simulink model "circuitTestSimulink_MDKTemplate_3DElectrical"  (R2024a)
settings: Solver=VariableStepAuto  StartTime=0.0  StopTime=1100e-9  FixedStep=1e-12  MaxStep=1e-10  RelTol=1e-2
undefined symbols (not defined in the file or in its folder): FMIKit
libraries: fl_lib x16, nesl_utility x10, ee_lib x4
settings Model: Creator=ezzbj2  LastModifiedBy=ezzbj2
settings SolverCC: ShapePreserveControl=EnableAll  ZeroCrossAlgorithm=Adaptive
settings RTWCC: GPUComputeCapability=3.5

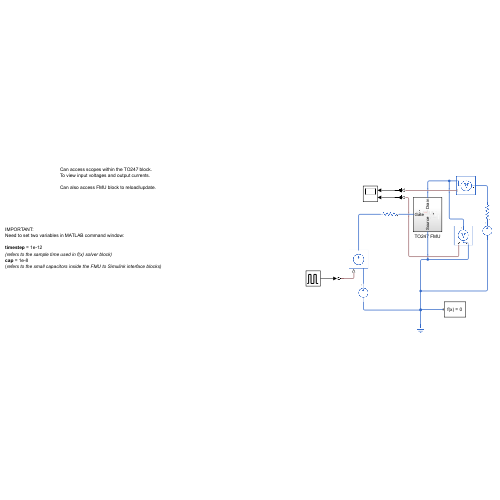
[thumbnail: Simulink's stored preview of the top-level diagram]
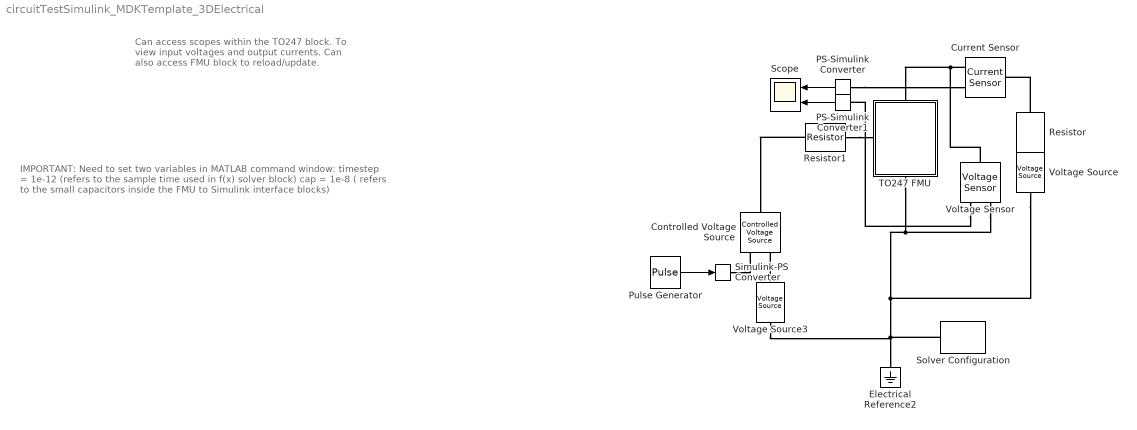
== system circuitTestSimulink_MDKTemplate_3DElectrical ==
  note: Can access scopes within the TO247 block.
      | To view input voltages and output currents.
      |
      | Can also access FMU block to reload/update.
  note: IMPORTANT:
      | Need to set two variables in MATLAB command window:
      |
      | timestep = 1e-12
      | (refers to the sample time used in f(x) solver block)
      | cap = 1e-8
      | ( refers to the small capacitors inside the FMU to Simulink interface blocks)
  Controlled Voltage Source : fl_lib/Electrical/Electrical Sources/Controlled Voltage Source
  Current Sensor : fl_lib/Electrical/Electrical Sensors/Current Sensor
  Electrical Reference2 : fl_lib/Electrical/Electrical Elements/Electrical Reference
  PS-Simulink Converter : nesl_utility/PS-Simulink Converter  PhysicalDomain=network_engine_domain  SubClassName=ps_output  LeftPortType=input  RightPortType=output  PseudoPeriodic=off  Frequencies=[]  VectorFormat=inherit  Unit=inherit  AffineConversion=off
  PS-Simulink Converter1 : nesl_utility/PS-Simulink Converter  PhysicalDomain=network_engine_domain  SubClassName=ps_output  LeftPortType=input  RightPortType=output  PseudoPeriodic=off  Frequencies=[]  VectorFormat=inherit  Unit=inherit  AffineConversion=off
  Pulse Generator : DiscretePulseGenerator  PulseType=Time based  Amplitude=15  Period=1000e-9  PulseWidth=50
  Resistor : ee_lib/Passive/Resistor  R=10 Ohm  enable_R_tol=ee.enum.toleranceApplication.none  R_tol=5  tol_distribution=ee.enum.toleranceDistribution.uniform  nSigma=4  enable_operating_limits=ee.enum.enable.no  operating_limit_action=ee.enum.passive.reportOpLim.warn  power_rating=1 W  max_working_voltage=100 V  enable_faults=ee.enum.enable.no  fault_action=simscape.enum.assert.action.none  R_faulted=inf Ohm  fault_trigger=ee.enum.faults.faultTrigger.temporal  t_fault=1 s  max_permissible_current=1 A  t_fail_on_current=1 s  noise_mode=ee.enum.sources.noise.Disabled  Tdevice=25 degC  sample_time=1e-3 s  repeatability=ee.enum.ic.repeatability.notRepeatable  user_seed=0  auto_seed=3499211588  faulted_specify=off  faulted_priority=None  faulted=0  power_derating_T1=70 degC  power_derating_T2=155 degC  operating_temperature_range_vec=[-50, 150] degC  alpha=3.93e-3 1/K  Tmeas=25 degC  thermal_mass=100 J/K  temperature_specify=off  temperature_priority=High  temperature=298.15 K  temperature_nominal_specify=off  temperature_nominal_value=1  temperature_nominal_unit=K
  Resistor1 : ee_lib/Passive/Resistor  R=2 Ohm  enable_R_tol=ee.enum.toleranceApplication.none  R_tol=5  tol_distribution=ee.enum.toleranceDistribution.uniform  nSigma=4  enable_operating_limits=ee.enum.enable.no  operating_limit_action=ee.enum.passive.reportOpLim.warn  power_rating=1 W  max_working_voltage=100 V  enable_faults=ee.enum.enable.no  fault_action=simscape.enum.assert.action.none  R_faulted=inf Ohm  fault_trigger=ee.enum.faults.faultTrigger.temporal  t_fault=1 s  max_permissible_current=1 A  t_fail_on_current=1 s  noise_mode=ee.enum.sources.noise.Disabled  Tdevice=25 degC  sample_time=1e-3 s  repeatability=ee.enum.ic.repeatability.notRepeatable  user_seed=0  auto_seed=3499211588  faulted_specify=off  faulted_priority=None  faulted=0  power_derating_T1=70 degC  power_derating_T2=155 degC  operating_temperature_range_vec=[-50, 150] degC  alpha=3.93e-3 1/K  Tmeas=25 degC  thermal_mass=100 J/K  temperature_specify=off  temperature_priority=High  temperature=298.15 K  temperature_nominal_specify=off  temperature_nominal_value=1  temperature_nominal_unit=K
  Scope : Scope  NumInputPorts=2
  Simulink-PS Converter : nesl_utility/Simulink-PS Converter  PhysicalDomain=network_engine_domain  SubClassName=ps_input  LeftPortType=input  RightPortType=output  PseudoPeriodic=off  Frequencies=[]  NoiseDistribution=none  NoiseParameters=[]  Unit=1  AffineConversion=off  FilteringAndDerivatives=provide  SimscapeFilterOrder=1  InputFilterTimeConstant=0.001  UdotUserProvided=0
  Solver Configuration : nesl_utility/Solver Configuration  PhysicalDomain=network_engine_domain  SubClassName=solver  LeftPortType=input  RightPortType=generic  Tones=[]  Harmonics=[]  SimulateNoise=off  Profile=off  UseLocalSampling=off  EnableSwitchedLinearOptims=on  FrequencyDomain=off  UseCCode=off  RelTol=0.001  AbsTol=0.001  MinStep=1e-09  ToWorkspace=off  RevertToSquareIcSolve=off  NumHomotopyIterations=100  PhasorMode=off  PhasorModeNumHarmonics=1  ConsistencySolver=NEWTON_XTOL_AFTER_FTOL  IndexReductionMethod=None  DoDC=on  ResidualTolerance=1e-09  ConsistencyTolSource=GLOBAL  ConsistencyAbsTol=0.001  ConsistencyRelTol=0.001  ConsistencyTolFactor=0.001  UseLocalSolver=off  LocalSolverChoice=NE_BACKWARD_EULER_ADVANCER  ResolveIndetEquations=on  FunctionEvalNumThread=1  LocalSolverSampleTime=timestep  DoFixedCost=off  MaxNonlinIter=30  MaxModeIter=2  ComputeImpulses=on  ImpulseIterations=2  LinearAlgebra=auto  LinearAlgebraNumThread=0  EquationFormulation=NE_TIME_EF  DelaysMemoryBudget=1024  AutomaticFiltering=off  FilteringTimeConstant=0.001  PartitionStorageMethod=EXHAUSTIVE  PartitionMemoryBudget=1024  PartitionMethod=ROBUST  MultibodyUseLocalSolver=off  MultibodyLocalSolverChoice=ODE1  MultibodyLocalSolverSampleTime=0.001
  TO247 FMU : Subsystem
      settings: PortSchema="{\"entries\":[{\"content\":{\"sides\":[{\"content\":{\"connectorIds\":[\"LConn1\"]},\"type\":\"ConnectorPlacement.EquallySpacedRectSide\",\"uuid\":\"1a7c621a-b2c4-44d6-8085-8acdfe65af3e\"},{\"content\":{\"side\":\"RIGHT\"},\"type\":\"ConnectorPlacement.EquallySpacedRectSide\",\"uuid\":\"009b5a79-97ab-42cc-83a0-e109b769c9f7\"},{\"content\":{\"connectorIds\":[\"LConn2\"],\"side\":\"TOP\"},\"type\":\"ConnectorPlacement.EquallySpacedRectSide\",\"uuid\":\"b2698f3e-d975-41db-922f-800e4c377170\"},{\"content\":{\"connectorIds\":[\"RConn1\"],\"side\":\"BOTTOM\"},\"type\":\"ConnectorPlacement.EquallySpacedRectSide\",\"uuid\":\"c87b7d4f-b69b-4cab-ae10-03d23c792008\"}]},\"type\":\"ConnectorPlacement.EquallySpacedConnector\",\"uuid\":\"776127ee-5564-4d8f-a192-88fd759918ca\"}],\"packageUris\":[\"http://schema.mathworks.com/mf0/Connector/R2020b\"],\"version\":\"1.0\"}"
  Voltage Sensor : fl_lib/Electrical/Electrical Sensors/Voltage Sensor
  Voltage Source : ee_lib/Sources/Voltage Source  dc_voltage=100 V  ac_voltage=0 V  ac_shift=0 rad  ac_frequency=60 Hz  noise_mode=ee.enum.sources.noise.Disabled  PSD=0 V^2/Hz  sample_time=1e-3 s  repeatability=ee.enum.sources.repeatability.NotRepeatable  user_seed=0  auto_seed=3890346746  i_specify=off  i_priority=None  i=0 A  i_nominal_specify=off  i_nominal_value=1  i_nominal_unit=A  v_specify=off  v_priority=None  v=0 V  v_nominal_specify=off  v_nominal_value=1  v_nominal_unit=V
  Voltage Source3 : ee_lib/Sources/Voltage Source  dc_voltage=0 V  ac_voltage=0 V  ac_shift=0 rad  ac_frequency=60 Hz  noise_mode=ee.enum.sources.noise.Disabled  PSD=0 V^2/Hz  sample_time=1e-3 s  repeatability=ee.enum.sources.repeatability.NotRepeatable  user_seed=0  auto_seed=3499211588  i_specify=off  i_priority=None  i=0 A  i_nominal_specify=off  i_nominal_value=1  i_nominal_unit=A  v_specify=off  v_priority=None  v=0 V  v_nominal_specify=off  v_nominal_value=1  v_nominal_unit=V
  wires:
  PS-Simulink Converter/1 -> Scope/1
  PS-Simulink Converter1/1 -> Scope/2
  Pulse Generator/1 -> Simulink-PS Converter/1
  connections:
  TO247 FMU/RConn1 -- Voltage Source/RConn1 -- Voltage Source3/RConn1 -- Electrical Reference2/LConn1 -- Solver Configuration/RConn1 -- Voltage Sensor/RConn2
  Current Sensor/RConn2 -- Voltage Sensor/LConn1 -- TO247 FMU/LConn2
  PS-Simulink Converter/LConn1 -- Current Sensor/RConn1
  Simulink-PS Converter/RConn1 -- Controlled Voltage Source/RConn1
  Voltage Source3/LConn1 -- Controlled Voltage Source/RConn2
  Voltage Sensor/RConn1 -- PS-Simulink Converter1/LConn1
  Resistor/RConn1 -- Voltage Source/LConn1
  Resistor/LConn1 -- Current Sensor/LConn1
  Resistor1/LConn1 -- TO247 FMU/LConn1
  Resistor1/RConn1 -- Controlled Voltage Source/LConn1

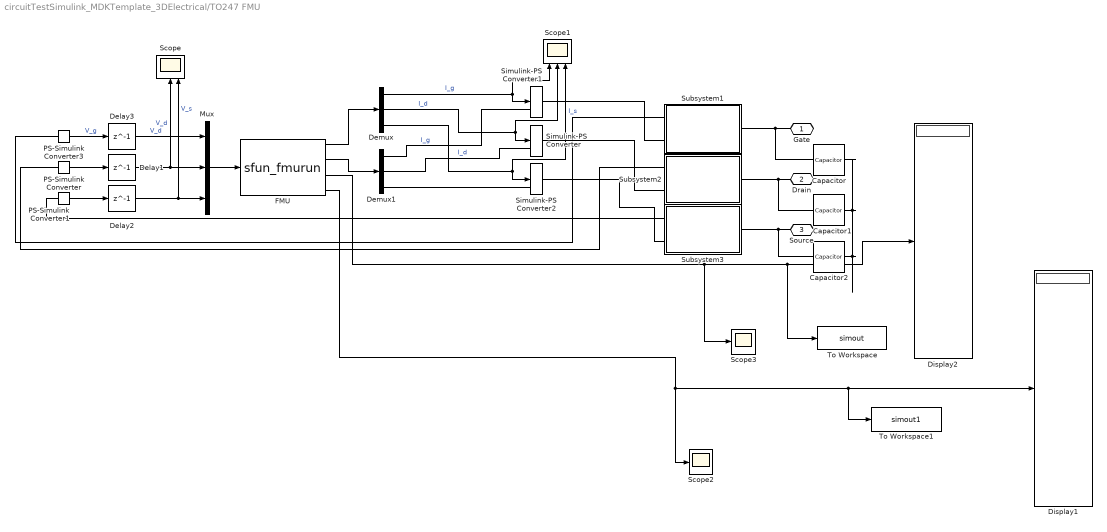
== system circuitTestSimulink_MDKTemplate_3DElectrical/TO247 FMU ==
  Capacitor : fl_lib/Electrical/Electrical Elements/Capacitor  c=1e-14 F  r=1e-6 Ohm  g=0 1/Ohm  i_specify=off  i_priority=None  i=0 A  i_nominal_specify=off  i_nominal_value=1  i_nominal_unit=A  v_specify=off  v_priority=None  v=0 V  v_nominal_specify=off  v_nominal_value=1  v_nominal_unit=V  vc_specify=off  vc_priority=High  vc=0 V  vc_nominal_specify=off  vc_nominal_value=1  vc_nominal_unit=V
  Capacitor1 : fl_lib/Electrical/Electrical Elements/Capacitor  c=1e-14 F  r=1e-6 Ohm  g=0 1/Ohm  i_specify=off  i_priority=None  i=0 A  i_nominal_specify=off  i_nominal_value=1  i_nominal_unit=A  v_specify=off  v_priority=None  v=0 V  v_nominal_specify=off  v_nominal_value=1  v_nominal_unit=V  vc_specify=off  vc_priority=High  vc=0 V  vc_nominal_specify=off  vc_nominal_value=1  vc_nominal_unit=V
  Capacitor2 : fl_lib/Electrical/Electrical Elements/Capacitor  c=1e-14 F  r=1e-6 Ohm  g=0 1/Ohm  i_specify=off  i_priority=None  i=0 A  i_nominal_specify=off  i_nominal_value=1  i_nominal_unit=A  v_specify=off  v_priority=None  v=0 V  v_nominal_specify=off  v_nominal_value=1  v_nominal_unit=V  vc_specify=off  vc_priority=High  vc=0 V  vc_nominal_specify=off  vc_nominal_value=1  vc_nominal_unit=V
  Delay1 : Delay  DelayLength=1
  Delay2 : Delay  DelayLength=1
  Delay3 : Delay  DelayLength=1
  Demux : Demux  Outputs=3
  Demux1 : Demux  Outputs=3
  Display1 : Display
  Display2 : Display
  FMU : S-Function  LoadFcn=FMIKit.setSFunctionParameters(gcb)  FunctionName=sfun_fmurun  Parameters=3.0 0 '{D773325B-AB94-4630-BF85-643EB24FCB80}' 'MDKCircuit_3DElectrical' FMIKit.getUnzipDirectory(gcb) 0 0 0 '' FMIKit.getSolverRelativeTolerance(bdroot(gcb)) -1 0 12 0 0 [3] [1.0] [2] [9] [3 3 16 12] [2 2 2 2] [10 24 13 11]  SFunctionDeploymentMode=off  EnableBusSupport=off
      settings: DeleteFcn=FMIKit.closeBlockDialog(gcbh)  ModelCloseFcn=FMIKit.closeBlockDialog(gcbh)  DestroyFcn=FMIKit.closeBlockDialog(gcbh)  OpenFcn=FMIKit.showBlockDialog(gcbh);  CloseFcn=FMIKit.closeBlockDialog(gcbh)  ParentCloseFcn=FMIKit.closeBlockDialog(gcbh)
      mask Help: eval('FMIKit.showBlockDialogHelp();')
      mask Display:
      | port_label('input', 1, 'u');
      | port_label('output', 1, 'y');
      | port_label('output', 2, 'dy');
      | port_label('output', 3, 'x_a');
      | port_label('output', 4, 'x_d');
  Mux : Mux  Inputs=3
  PS-Simulink Converter : nesl_utility/PS-Simulink Converter  PhysicalDomain=network_engine_domain  SubClassName=ps_output  LeftPortType=input  RightPortType=output  PseudoPeriodic=off  Frequencies=[]  VectorFormat=inherit  Unit=inherit  AffineConversion=off
  PS-Simulink Converter1 : nesl_utility/PS-Simulink Converter  PhysicalDomain=network_engine_domain  SubClassName=ps_output  LeftPortType=input  RightPortType=output  PseudoPeriodic=off  Frequencies=[]  VectorFormat=inherit  Unit=inherit  AffineConversion=off
  PS-Simulink Converter3 : nesl_utility/PS-Simulink Converter  PhysicalDomain=network_engine_domain  SubClassName=ps_output  LeftPortType=input  RightPortType=output  PseudoPeriodic=off  Frequencies=[]  VectorFormat=inherit  Unit=inherit  AffineConversion=off
  Scope : Scope  NumInputPorts=3
  Scope1 : Scope  NumInputPorts=3
  Scope2 : Scope
  Scope3 : Scope
  Simulink-PS Converter : nesl_utility/Simulink-PS Converter  PhysicalDomain=network_engine_domain  SubClassName=ps_input  LeftPortType=input  RightPortType=output  PseudoPeriodic=off  Frequencies=[]  NoiseDistribution=none  NoiseParameters=[]  Unit=1  AffineConversion=off  FilteringAndDerivatives=filter  SimscapeFilterOrder=1  InputFilterTimeConstant=1e-9  UdotUserProvided=1
  Simulink-PS Converter1 : nesl_utility/Simulink-PS Converter  PhysicalDomain=network_engine_domain  SubClassName=ps_input  LeftPortType=input  RightPortType=output  PseudoPeriodic=off  Frequencies=[]  NoiseDistribution=none  NoiseParameters=[]  Unit=1  AffineConversion=off  FilteringAndDerivatives=filter  SimscapeFilterOrder=1  InputFilterTimeConstant=1e-9  UdotUserProvided=1
  Simulink-PS Converter2 : nesl_utility/Simulink-PS Converter  PhysicalDomain=network_engine_domain  SubClassName=ps_input  LeftPortType=input  RightPortType=output  PseudoPeriodic=off  Frequencies=[]  NoiseDistribution=none  NoiseParameters=[]  Unit=1  AffineConversion=off  FilteringAndDerivatives=filter  SimscapeFilterOrder=1  InputFilterTimeConstant=1e-9  UdotUserProvided=1
  Subsystem1 : Subsystem
  Subsystem2 : Subsystem
  Subsystem3 : Subsystem
  To Workspace : ToWorkspace  VariableName=simout  SaveFormat=Timeseries  SampleTime=-1
  To Workspace1 : ToWorkspace  VariableName=simout1  SaveFormat=Timeseries  SampleTime=-1
  Gate : PMIOPort  Side=Left
  Drain : PMIOPort  Port=2  Side=Left
  Source : PMIOPort  Port=3  Side=Right
  wires:
  PS-Simulink Converter1/1 -> Delay2/1
  Delay2/1 -> Scope/3, Mux/3  "V_s"
  Delay1/1 -> Scope/2, Mux/2  "V_d"
  PS-Simulink Converter/1 -> Delay1/1
  FMU/3 -> Scope3/1, To Workspace/1, Display2/1
  FMU/4 -> Scope2/1, To Workspace1/1, Display1/1
  Delay3/1 -> Mux/1  "V_d"
  PS-Simulink Converter3/1 -> Delay3/1  "V_g"
  Mux/1 -> FMU/1
  FMU/1 -> Demux/1
  FMU/2 -> Demux1/1
  Demux/1 -> Simulink-PS Converter1/1, Scope1/1  "I_g"
  Demux/2 -> Scope1/2, Simulink-PS Converter/1  "I_d"
  Demux/3 -> Simulink-PS Converter2/1, Scope1/3  "I_s"
  Demux1/1 -> ?  "I_g"
  Demux1/2 -> ?  "I_d"
  Demux1/3 -> ?
  connections:
  Simulink-PS Converter1/RConn1 -- Subsystem1/LConn2
  Subsystem2/LConn1 -- PS-Simulink Converter/LConn1
  PS-Simulink Converter3/LConn1 -- Subsystem1/LConn1
  Subsystem3/LConn1 -- PS-Simulink Converter1/LConn1
  Subsystem2/LConn2 -- Simulink-PS Converter/RConn1
  Subsystem3/LConn2 -- Simulink-PS Converter2/RConn1
  Gate/RConn1 -- Capacitor/LConn1 -- Subsystem1/RConn1
  Drain/RConn1 -- Capacitor1/LConn1 -- Subsystem2/RConn1
  Source/RConn1 -- Capacitor2/LConn1 -- Subsystem3/RConn1
  Capacitor2/RConn1 -- Capacitor1/RConn1 -- Capacitor/RConn1

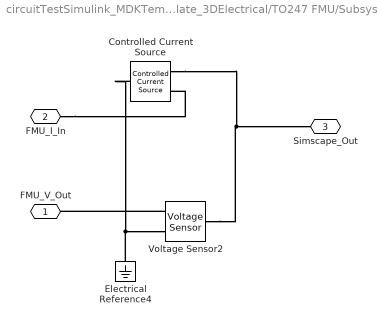
== system circuitTestSimulink_MDKTemplate_3DElectrical/TO247 FMU/Subsystem1 ==
  Controlled Current Source : fl_lib/Electrical/Electrical Sources/Controlled Current Source
  Electrical Reference4 : fl_lib/Electrical/Electrical Elements/Electrical Reference
  Voltage Sensor2 : fl_lib/Electrical/Electrical Sensors/Voltage Sensor
  FMU_V_Out : PMIOPort  Side=Left
  FMU_I_In : PMIOPort  Port=2  Side=Left
  Simscape_Out : PMIOPort  Port=3  Side=Right
  connections:
  Voltage Sensor2/RConn1 -- FMU_V_Out/RConn1
  FMU_I_In/RConn1 -- Controlled Current Source/RConn1
  Electrical Reference4/LConn1 -- Controlled Current Source/LConn1 -- Voltage Sensor2/RConn2
  Voltage Sensor2/LConn1 -- Controlled Current Source/RConn2 -- Simscape_Out/RConn1

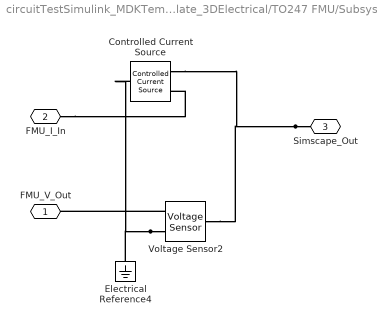
== system circuitTestSimulink_MDKTemplate_3DElectrical/TO247 FMU/Subsystem2 ==
  Controlled Current Source : fl_lib/Electrical/Electrical Sources/Controlled Current Source
  Electrical Reference4 : fl_lib/Electrical/Electrical Elements/Electrical Reference
  Voltage Sensor2 : fl_lib/Electrical/Electrical Sensors/Voltage Sensor
  FMU_V_Out : PMIOPort  Side=Left
  FMU_I_In : PMIOPort  Port=2  Side=Left
  Simscape_Out : PMIOPort  Port=3  Side=Right
  connections:
  Voltage Sensor2/RConn1 -- FMU_V_Out/RConn1
  FMU_I_In/RConn1 -- Controlled Current Source/RConn1
  Voltage Sensor2/RConn2 -- Electrical Reference4/LConn1 -- Controlled Current Source/LConn1
  Simscape_Out/RConn1 -- Voltage Sensor2/LConn1 -- Controlled Current Source/RConn2

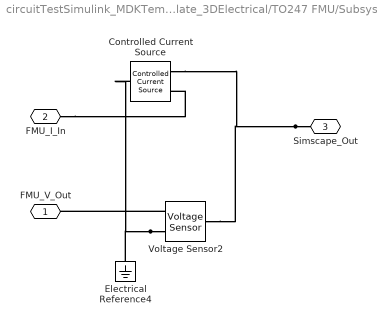
== system circuitTestSimulink_MDKTemplate_3DElectrical/TO247 FMU/Subsystem3 ==
  Controlled Current Source : fl_lib/Electrical/Electrical Sources/Controlled Current Source
  Electrical Reference4 : fl_lib/Electrical/Electrical Elements/Electrical Reference
  Voltage Sensor2 : fl_lib/Electrical/Electrical Sensors/Voltage Sensor
  FMU_V_Out : PMIOPort  Side=Left
  FMU_I_In : PMIOPort  Port=2  Side=Left
  Simscape_Out : PMIOPort  Port=3  Side=Right
  connections:
  Voltage Sensor2/RConn1 -- FMU_V_Out/RConn1
  FMU_I_In/RConn1 -- Controlled Current Source/RConn1
  Voltage Sensor2/RConn2 -- Electrical Reference4/LConn1 -- Controlled Current Source/LConn1
  Simscape_Out/RConn1 -- Voltage Sensor2/LConn1 -- Controlled Current Source/RConn2
